simulink model "GCU_Model_genCode"  (R2018a)
settings: Solver=FixedStepDiscrete  StartTime=0.0  StopTime=20  FixedStep=0.0001  RelTol=1e-3  EnableMultiTasking=on
undefined symbols (not defined in the file): ConversionGainVector, ConversionOffsetVector, VoltageGainVector, VoltageOffsetVector
libraries: canLib x5, simulink x5, uartLib x2, utilityLib x1, clutchMotorLib x1, efiLib x1, engineControlLib x1, cstblocks x1, gearMotorLib x1
(part 3 of 3)

== stateflow chart GCU_Model_genCode/CAN_Send/CAN_id ==
  (default) -> (junction 1) : {gcu_traction_limiter_loil_efi_id = GCU_TRACTION_LIMITER_LOIL_EFI_ID;
      |  gcu_clutch_mode_map_sw_id = GCU_CLUTCH_MODE_MAP_SW_ID;
      |  gcu_traction_limiter_autog_acc_sw_id = GCU_TRACTION_LIMITER_AUTOG_ACC_SW_ID;
      |  gcu_debug_1_id = GCU_DEBUG_1_ID;
      |  gcu_debug_2_id = GCU_DEBUG_2_ID;}
  (junction 1) -> (junction 12) [order 1] : [counter3 >= 100]
  (junction 1) -> (junction 16) [order 2]
  (junction 12) -> (junction 14) : {send(send1Hz);
      |   counter3 = 0;}
  (junction 16) -> (junction 14) [order 1] : [counter2 >= 10 ]
  (junction 16) -> (junction 28) [order 2]
  (junction 14) -> (junction 23) : {send(send10Hz);
      |  counter2 = 0;}
  (junction 28) -> (junction 23)
  (junction 23) -> (junction 26) : {send(send100Hz);
      |  counter2++;
      |  counter3++;}
  data: gcu_traction_limiter_loil_efi_id output uint16 size=1; gcu_clutch_mode_map_sw_id output uint16 size=1; gcu_traction_limiter_autog_acc_sw_id output uint16 size=1; gcu_debug_1_id output uint16 size=1; gcu_debug_2_id output uint16 size=1; counter3 local uint8 =uint8(0); counter1 local uint8 =uint8(0); counter2 local uint8 =uint8(0)
  events: send100Hz output FUNCTION_CALL_EVENT; send10Hz output FUNCTION_CALL_EVENT; send1Hz output FUNCTION_CALL_EVENT

== stateflow chart GCU_Model_genCode/EEPROM/EEPROM_Load_Buffer ==
  settings: executeAtInitialization=1
  state updateBuffer [function]
    (default) -> (junction 12)
    (junction 12) -> (junction 14) [order 1] : [lastInsertedIndex >=20]
    (junction 12) -> (junction 19) [order 2] : {lastInsertedIndex = lastInsertedIndex + 1;}
    (junction 14) -> (junction 16) : {lastInsertedIndex = 1;}
    (junction 19) -> (junction 16)
    (junction 16) -> (junction 22) : {requestBuffer(lastInsertedIndex).operation = inputRequest.operation;
        |  requestBuffer(lastInsertedIndex).page = inputRequest.page;
        |  requestBuffer(lastInsertedIndex).cell = inputRequest.cell;
        |  requestBuffer(lastInsertedIndex).dataSize = inputRequest.dataSize;
        |  requestBuffer(lastInsertedIndex).data = inputRequest.data;}
  (default) -> (junction 52) : {updateBuffer();}
  data: inputRequest input Bus: eepromRequest size=1; requestBuffer output Bus: eepromRequest size=[1,20]; lastInsertedIndex output double =1
  events: serialRequest input FUNCTION_CALL_EVENT

== stateflow chart GCU_Model_genCode/EEPROM/EEPROM_OutputRequest ==
  settings: executeAtInitialization=1
  state createRequest(operation, page, cell, dataSize, tempData) [function]
    (default) -> (junction 77) : {outputRequest.operation = operation;
        |  outputRequest.page = page;
        | outputRequest.cell = cell;
        | outputRequest.dataSize = dataSize;
        | outputRequest.data = tempData;}
  state LOAD_TO_EEPROM
    state index = shiftArray(array, nValues) [function]
      (default) -> (junction 106) : {tempShiftedArray = uint8(zeros(1,50));}
      (junction 107) -> (junction 105) [order 1] : [index <= nValues]
      (junction 106) -> (junction 107) : {index=1;}
      (junction 105) -> (junction 108) : {tempShiftedArray(2*index - 1) = uint8(bitshift(array(index), -8));
          |  tempShiftedArray(2*index) = uint8(bitand(uint16(array(index)),uint16(255)));}
      (junction 108) -> (junction 107) : {index=index+1;}
      (junction 107) -> (junction 109) [order 2]
    state extractValues(count) [function]
      (default) -> (junction 124)
      (junction 125) -> (junction 123) [order 1] : [index<= 16]
      (junction 123) -> (junction 126) : {newData(index) = tempShiftedArray(index+16*count);}
      (junction 124) -> (junction 125) : {index=1;}
      (junction 126) -> (junction 125) : {index=index+1;}
      (junction 125) -> (junction 127) [order 2]
    state FIRST_BYTE
      en:
      newData(1) = uint8(eepromConstants.USED_EEPROM);
      createRequest(uint8('W'), uint8(0),uint8(0), uint8(1), uint8(newData));
      send(evaluateRequest);
    state ANTI_STALL_PARAMETERS
      entry:
      shiftArray(antiStallInitialParameters, double(eepromConstants.ANTI_STALL_PAR_NUM));
      during: %!!~NON METTERE ENTRY SE NO EEPROM NON HA DELAY
      extractValues(counter);
      createRequest(uint8('W'), uint8(counter+11),uint8(0),uint8(16),uint8(newData));
      send(evaluateRequest);
      counter = counter + 1;
    state GEARSHIFT_TIMINGS
      entry:
      shiftArray(gearshiftInitialTimings, double(eepromConstants.GEARSHIFT_NUM) );
      entry,during:
      extractValues(counter);
      createRequest(uint8('W'), uint8(counter+1), uint8(0), uint8(16), uint8(newData));
      send(evaluateRequest);
      counter = counter + 1;
      %dataDebug = newData;
    state AUTOX_PARAMETERS
      entry:
      shiftArray(autoXInitialParameters, double(eepromConstants.AUTOX_PAR_NUM));
      during: %!!~NON METTERE ENTRY SE NO EEPROM NON HA DELAY
      extractValues(counter);
      createRequest(uint8('W'), uint8(counter+8),uint8(0),uint8(16),uint8(newData));
      send(evaluateRequest);
      counter = counter + 1;
    state ACC_PARAMETERS
      entry:
      shiftArray(accInitialParameters, double(eepromConstants.ACC_PAR_NUM));
      during: %!!~NON METTERE ENTRY SE NO EEPROM NON HA DELAY
      extractValues(counter);
      createRequest(uint8('W'), uint8(counter+5),uint8(0),uint8(16),uint8(newData));
      send(evaluateRequest);
      counter = counter + 1;
      %dataDebug = newData;
    (default) -> FIRST_BYTE : {counter = 0;}
    FIRST_BYTE -> LOAD_TO_EEPROM.GEARSHIFT_TIMINGS
    LOAD_TO_EEPROM.ACC_PARAMETERS -> LOAD_TO_EEPROM.AUTOX_PARAMETERS : [counter >=2]{counter = 0}
    LOAD_TO_EEPROM.AUTOX_PARAMETERS -> LOAD_TO_EEPROM.ANTI_STALL_PARAMETERS : [counter >=2]{counter = 0}
    LOAD_TO_EEPROM.GEARSHIFT_TIMINGS -> LOAD_TO_EEPROM.ACC_PARAMETERS : [counter >= 3]{ counter = 0;}
  state INIT
  state testIndex [function]
    (default) -> (junction 183)
    (junction 183) -> (junction 186) [order 1] : [lastInsertedIndex ~= lastEvaluatedIndex]
    (junction 183) -> (junction 188) [order 2]
    (junction 186) -> (junction 184) : {updateOutput();
        |  send(evaluateRequest);}
    (junction 184) -> (junction 230) [order 1] : [outputRequest.operation == uint8('W')]
    (junction 184) -> (junction 234) [order 2]
    (junction 230) -> (junction 232) : {reloadFlag = 1;}
  state LOAD_FROM_EEPROM
    state GEARSHIFT_TIMINGS
      entry,during:
      createRequest(uint8('L'), uint8(counter+1), uint8(0), uint8(16), uint8(zeros(1,16)));
      send(evaluateRequest);
      counter = counter + 1;
    state ACC_PARAMETERS
      entry:
      counter = 4;
      during:
      createRequest(uint8('L'), uint8(counter+1), uint8(0), uint8(16), uint8(zeros(1,16)));
      send(evaluateRequest);
      counter = counter +1;
    state AUTOX_PARAMETERS
      entry:
      counter = 7;
      during:
      createRequest(uint8('L'), uint8(counter+1), uint8(0), uint8(16), uint8(zeros(1,16)));
      send(evaluateRequest);
      counter = counter +1;
    state ANTI_STALL_PARAMETERS
      entry:
      counter = 10;
      during:
      createRequest(uint8('L'), uint8(counter+1), uint8(0), uint8(16), uint8(zeros(1,16)));
      send(evaluateRequest);
      counter = counter +1;
    (default) -> LOAD_FROM_EEPROM.GEARSHIFT_TIMINGS : {counter = 0}
    LOAD_FROM_EEPROM.GEARSHIFT_TIMINGS -> LOAD_FROM_EEPROM.ACC_PARAMETERS : [counter>=3]
    LOAD_FROM_EEPROM.ACC_PARAMETERS -> LOAD_FROM_EEPROM.AUTOX_PARAMETERS : [counter>=6]
    LOAD_FROM_EEPROM.AUTOX_PARAMETERS -> LOAD_FROM_EEPROM.ANTI_STALL_PARAMETERS : [counter>=9]
  state SERIAL_UPDATES [group]
    note: DA CAPIRE COME FUNZIONA PERCHE' LA WRITE E' SU INTERRUPT
    state EVALUATE_SERIAL
      during:
      testIndex();
    state RELOAD
      during:
      reloadFlag = 0;
      outputRequest.operation = uint8('L');
      outputRequest.cell = uint8(0);
      outputRequest.dataSize = uint8(16);
      send(evaluateRequest);
    EVALUATE_SERIAL -> RELOAD : [reloadFlag == 1 && writeResult ~= HAL_ERROR]
    RELOAD -> EVALUATE_SERIAL : [reloadFlag == 0]
  state updateOutput [function]
    (default) -> (junction 30)
    (junction 30) -> (junction 31) [order 1] : [lastEvaluatedIndex >=20]
    (junction 30) -> (junction 32) [order 2] : {lastEvaluatedIndex = lastEvaluatedIndex + 1;}
    (junction 31) -> (junction 33) : {lastEvaluatedIndex = 1;}
    (junction 32) -> (junction 33)
    (junction 33) -> (junction 34) : {outputRequest.operation = requestBuffer(lastEvaluatedIndex).operation ;
        |  outputRequest.page = requestBuffer(lastEvaluatedIndex).page;
        |  outputRequest.cell = requestBuffer(lastEvaluatedIndex).cell;
        |  outputRequest.dataSize = requestBuffer(lastEvaluatedIndex).dataSize;
        |  outputRequest.data = requestBuffer(lastEvaluatedIndex).data;
        | }
  state ERROR
    (default) -> (junction 152) : {createRequest(uint8('E'), uint8(0), uint8(0), uint8(0), uint8(zeros(1,16)));
        |  send(evaluateRequest);}
  (default) -> INIT
  INIT -> (junction 57)
  LOAD_TO_EEPROM.ANTI_STALL_PARAMETERS -> LOAD_FROM_EEPROM : [counter>=1]{counter = 0;}
  (junction 57) -> LOAD_TO_EEPROM [order 1] : [eepromState == uint8(eepromConstants.NEW_EEPROM)]
  (junction 57) -> (junction 63) [order 2]
  (junction 63) -> LOAD_FROM_EEPROM [order 1] : [eepromState == uint8(eepromConstants.USED_EEPROM)]
  (junction 63) -> ERROR [order 2]
  LOAD_FROM_EEPROM.ANTI_STALL_PARAMETERS -> EVALUATE_SERIAL : [counter>= 11]
  ERROR -> EVALUATE_SERIAL
  data: operation function_input uint8; page function_input uint8; cell function_input uint8; dataSize function_input uint8; tempData function_input uint8 size=[1,16]; array function_input uint16; nValues function_input size=1; index function_output double; count function_input uint8; newData local uint8 size=[1,16] =uint8(zeros(1,16)); HAL_ERROR local uint8 =uint8(1); eepromState input; accInitialParameters input; autoXInitialParameters input; gearshiftInitialTimings input; antiStallInitialParameters input; writeResult input uint8; outputRequest output Bus: eepromRequest size=1; requestBuffer input Bus: eepromRequest size=[1,20]; lastInsertedIndex input double =1; lastEvaluatedIndex local =1; tempShiftedArray local uint8 size=[1,50] =uint8(zeros(1,50)); counter local uint8 =uint8(0); reloadFlag local =0
  events: trigger input FUNCTION_CALL_EVENT; evaluateRequest output FUNCTION_CALL_EVENT

== stateflow chart GCU_Model_genCode/EEPROM/Evaluate_Request/LoadFromEEPROM/updateValues ==
  state LOAD_TIMINGS [group]
    (junction 18) -> (junction 61) : {indexTemp = page*8-7;
        |  gearshiftTimings(indexTemp: indexTemp+7) = data_16bit;}
  state LOAD_ACC_PARAMETERS [group]
    (junction 31) -> (junction 64) : {indexTemp = (page-4)*8-7;
        | accParameters(indexTemp : indexTemp+7) = data_16bit;}
  state LOAD_AUTOX_PARAMETERS [group]
    (junction 79) -> (junction 81) : {indexTemp = (page-7)*8-7;
        |  autoXParameters(indexTemp : indexTemp+7) = data_16bit;}
  state LOAD_ANTI_STALL_PARAMETERS [group]
    (junction 92) -> (junction 96) : {indexTemp = (page-10)*8-7;
        |  antiStallParameters(indexTemp : indexTemp+7) = data_16bit;}
  (default) -> (junction 85)
  (junction 56) -> (junction 54) [order 1] : [index<=8]
  (junction 54) -> (junction 57) : {data_16bit(index) = bitshift(uint16(data_8bit(2*index-1)), 8) + uint16(data_8bit(2*index));}
  (junction 85) -> (junction 55) [order 1] : [loadResult ~= HAL_ERROR]
  (junction 85) -> (junction 87) [order 2]
  (junction 55) -> (junction 56) : {index=1;}
  (junction 57) -> (junction 56) : {index=index+1;}
  (junction 56) -> (junction 14) [order 2]
  (default) -> (junction 73) [commented out]
  (junction 74) -> (junction 72) [commented out] : [index<=8]
  (junction 72) -> (junction 75) [commented out] : {paramsArray(index) = }
  (junction 73) -> (junction 74) [commented out] : {index=1;}
  (junction 75) -> (junction 74) [commented out] : {index=index+1;}
  (junction 74) -> (junction 76) [commented out]
  (junction 14) -> (junction 18) [order 1] : [page == uint8(1) || page == uint8(2) || page == uint8(3)]
  (junction 14) -> (junction 29) [order 2]
  (junction 29) -> (junction 31) [order 1] : [page == uint8(5) || page == uint8(6)]
  (junction 29) -> (junction 33) [order 2]
  (junction 33) -> (junction 79) [order 1] : [page == uint8(8) || page == uint8(9)]
  (junction 33) -> (junction 37) [order 2]
  (junction 37) -> (junction 92) [order 1] : [page == uint8(11)]
  (junction 37) -> (junction 94) [order 2]
  data: loadResult input uint8; page input uint8; cell input uint8; dataSize input uint8; data_8bit input uint8 size=[1,16]; gearshiftTimings output uint16 size=[1,24] =uint16(zeros(1,24));; accParameters output uint16 size=[1,16] =uint16(zeros(1,16));; data_16bit local uint16 size=[1,8] =uint16(zeros(1,8)); index local; indexTemp local; autoXParameters output uint16 size=[1,16] =uint16(zeros(1,16));; HAL_ERROR local uint8 =uint8(1); antiStallParameters output uint16 size=[1,8] =uint16(zeros(1,8));

== stateflow chart GCU_Model_genCode/GCU_timer/Anti_Stall_System/antiStallLogic ==
  settings: executeAtInitialization=1
  state param = getAntiStallParam(index) [function]
    (default) -> (junction 55)
    (junction 55) -> (junction 56) : {param = antiStall_parameters[int32(index)]}
  state AntiStallActivate(Inport) [function]
  (default) -> (junction 7) : {antiStallState=0;}
  (junction 7) -> (junction 9) [order 1] : [enable == 1]
  (junction 7) -> (junction 25) [order 2]
  (junction 9) -> (junction 11) : {antiStallState=1;}
  (junction 11) -> (junction 13) [order 1] : [stop == 0]
  (junction 13) -> (junction 41) : {antiStallState=2;}
  (junction 11) -> (junction 27) [order 2] : {antiStallFb= ANTISTALL_OFF;
      | antiStallClutchVal = 0;}
  (junction 41) -> (junction 43) [order 1] : [currGear >= getAntiStallParam(anti_stall_params.GEAR_THRESHOLD)]
  (junction 41) -> (junction 46) [order 2]
  (junction 43) -> (junction 15) : {antiStallState=3;}
  (junction 15) -> (junction 17) [order 1] : [rpm <= getAntiStallParam(anti_stall_params.RPM_THRESHOLD)]
  (junction 15) -> (junction 28) [order 2]
  (junction 17) -> (junction 19) : {antiStallState=4;}
  (junction 19) -> (junction 21) [order 1] : [deltarpm <= -getAntiStallParam(anti_stall_params.RPM_DELTA_THRESHOLD)]
  (junction 19) -> (junction 29) [order 2]
  (junction 21) -> (junction 23) : {%send(antiStallActivate);
      |  AntiStallActivate(uint8(0));
      |  antiStallFb = ANTISTALL_ON;
      |   antiStallState=5;
      |   antiStallClutchVal = 100;}
  (junction 25) -> (junction 27)
  (junction 27) -> (junction 46)
  (junction 46) -> (junction 28)
  (junction 28) -> (junction 29)
  (junction 29) -> (junction 37)
  data: index function_input Enum: anti_stall_params size=1; param function_output int32 size=1; Inport function_input; enable input; stop input; antiStall_parameters input int32 size=[1,8]; rpm input; deltarpm input; antiStallFb output uint16 =uint16(0); currGear input; antiStallState output double; antiStallClutchVal output uint8 =uint8(0)
  events: antiStallActivate output FUNCTION_CALL_EVENT

== stateflow chart GCU_Model_genCode/Anti_Stall_Debug/AccelerationRoutine ==
  settings: executeAtInitialization=1
  state Wait
  state delay
    entry:
    count = 0;
    during:
    count = count + 1;
  state AntiStall
    entry:
    rpm = 20000;
    id = 773;
    firstInt = 1;
    during:
    rpm = rpm - 1000;
    secondInt = rpm;
  state checkGear [function]
    (default) -> (junction 55)
    (junction 55) -> (junction 57) [order 1] : [gearPin == 0 && lastGearPin ==1]
    (junction 55) -> (junction 61) [order 2]
    (junction 57) -> (junction 59) : {currGear = currGear + 1;}
    (junction 59) -> (junction 64)
    (junction 61) -> (junction 64)
    (junction 64) -> (junction 67) : {lastGearPin = gearPin}
  state clutch
    entry:
    id = 513;
    firstInt = 50;
  (default) -> Wait
  Wait -> delay
  delay -> AntiStall : [count == 50]
  AntiStall -> clutch : [rpm == 0]
  data: id output uint16; firstInt output uint16; secondInt output uint16 =uint16(0);; counter local; gearPin input uint8; lastGearPin local uint8 =uint8(0); message local =0; rpm local uint16; currGear local uint16 =uint16(0);; count local; thirdInt output uint16 =uint16(0);

== stateflow chart GCU_Model_genCode/GCU_timer/Anti_Stall_System/timeCounter ==
  (default) -> (junction 13)
  (junction 13) -> (junction 3) : {timeMs = timeMs + 1;}
  (junction 3) -> (junction 6) [order 1] : [rpmUpdateCounter ~= lastRPMUpdate]
  (junction 3) -> (junction 10) [order 2]
  (junction 6) -> (junction 8) : {deltaTime = timeMs;
      | timeMs = 0;
      |  lastRPMUpdate = rpmUpdateCounter;
      |  lastRPMValue = rpm;}
  data: rpmUpdateCounter input; lastRPMUpdate local uint8 =uint8(0); deltaTime output =0; timeMs local =0; lastRPMValue output uint16 =uint16(0); rpm input
